simulink model "all_in_one"  (R2022b)
settings: Solver=VariableStepAuto  StartTime=0.0  StopTime=10.0  RelTol=1e-3
settings Model: Creator=GROUP LAPTOPS  LastModifiedBy=GROUP LAPTOPS
settings OptimizationCC: DefaultParameterBehavior=Inlined  EnhancedBackFolding=on  PassReuseOutputArgsThreshold=0  OptimizeBlockOrder=speed  DifferentSizesBufferReuse=on  OptimizationCustomize=off
settings DebuggingCC: ParameterTunabilityLossMsg=error
settings HardwareCC: TargetBitPerPointer=64  TargetBitPerSizeT=64  TargetBitPerPtrDiffT=64  TargetLongLongMode=on  TargetIntDivRoundTo=Zero  TargetEndianess=LittleEndian  TargetWordSize=64  TargetHWDeviceType=MATLAB Host  ProdEqTarget=off
settings SFSimCC: MATLABDynamicMemAlloc=off
settings RTWCC: Description=Rapid Simulation Target  SystemTargetFile=rsim.tlc  TemplateMakefile=rsim_default_tmf  GenerateReport=on
settings CodeAppCC: ForceParamTrailComments=on  OperatorAnnotations=on
settings RSimTargetCC: TargetLangStandard=C99 (ISO)  OptimizeReductions=off

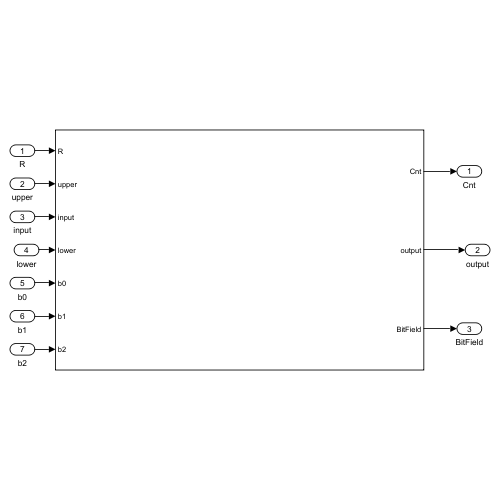
[thumbnail: Simulink's stored preview of the top-level diagram]
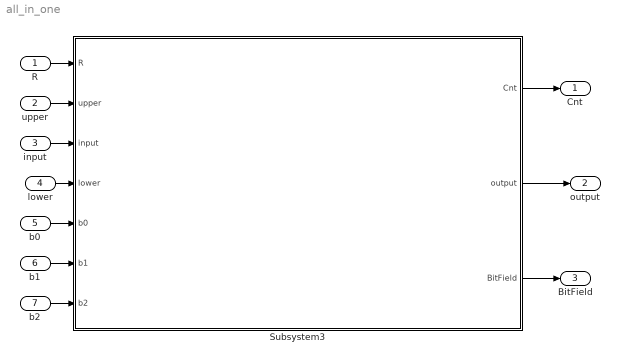
== system all_in_one ==
  R : Inport
  upper : Inport  Port=2
  input : Inport  Port=3
  lower : Inport  Port=4
  b0 : Inport  Port=5
  b1 : Inport  Port=6
  b2 : Inport  Port=7
  Subsystem3 : Subsystem
  Cnt : Outport
  output : Outport  Port=2
  BitField : Outport  Port=3
  wires:
  R/1 -> Subsystem3/1(R)
  upper/1 -> Subsystem3/2(upper)
  input/1 -> Subsystem3/3(input)
  lower/1 -> Subsystem3/4(lower)
  b2/1 -> Subsystem3/7(b2)
  b1/1 -> Subsystem3/6(b1)
  b0/1 -> Subsystem3/5(b0)
  Subsystem3/1(Cnt) -> Cnt/1
  Subsystem3/3(BitField) -> BitField/1
  Subsystem3/2(output) -> output/1

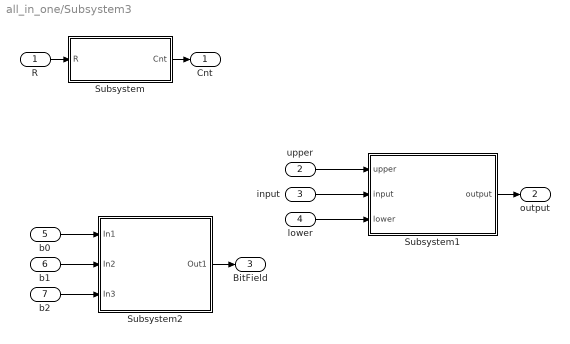
== system all_in_one/Subsystem3 ==
  R : Inport
  upper : Inport  Port=2
  input : Inport  Port=3
  lower : Inport  Port=4
  b0 : Inport  Port=5
  b1 : Inport  Port=6
  b2 : Inport  Port=7
  Subsystem : Subsystem
  Subsystem1 : Subsystem
  Subsystem2 : Subsystem
  Cnt : Outport
  output : Outport  Port=2
  BitField : Outport  Port=3
  wires:
  b0/1 -> Subsystem2/1(In1)
  Subsystem2/1(Out1) -> BitField/1
  upper/1 -> Subsystem1/1(upper)
  Subsystem1/1(output) -> output/1
  R/1 -> Subsystem/1(R)
  input/1 -> Subsystem1/2(input)
  Subsystem/1(Cnt) -> Cnt/1
  b1/1 -> Subsystem2/2(In2)
  b2/1 -> Subsystem2/3(In3)
  lower/1 -> Subsystem1/3(lower)

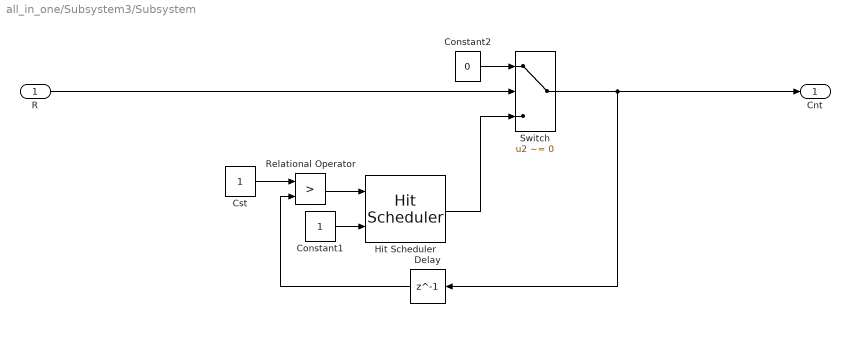
== system all_in_one/Subsystem3/Subsystem ==
  R : Inport
  Constant1 : Constant
  Constant2 : Constant  Value=0
  Cst : Constant
  Delay : Delay  DelayLength=1  InitialCondition=0
  Hit Scheduler : HitScheduler
  Relational Operator : RelationalOperator  Operator=>  OutDataTypeStr=boolean  RndMeth=Simplest  InputSameDT=off
  Switch : Switch  Criteria=u2 ~= 0  SaturateOnIntegerOverflow=off  InputSameDT=off
  Cnt : Outport
  wires:
  Relational Operator/1 -> Hit Scheduler/1
  Constant1/1 -> Hit Scheduler/2
  Switch/1 -> Cnt/1, Delay/1
  Delay/1 -> Relational Operator/2
  Cst/1 -> Relational Operator/1
  Constant2/1 -> Switch/1
  Hit Scheduler/1 -> Switch/3
  R/1 -> Switch/2

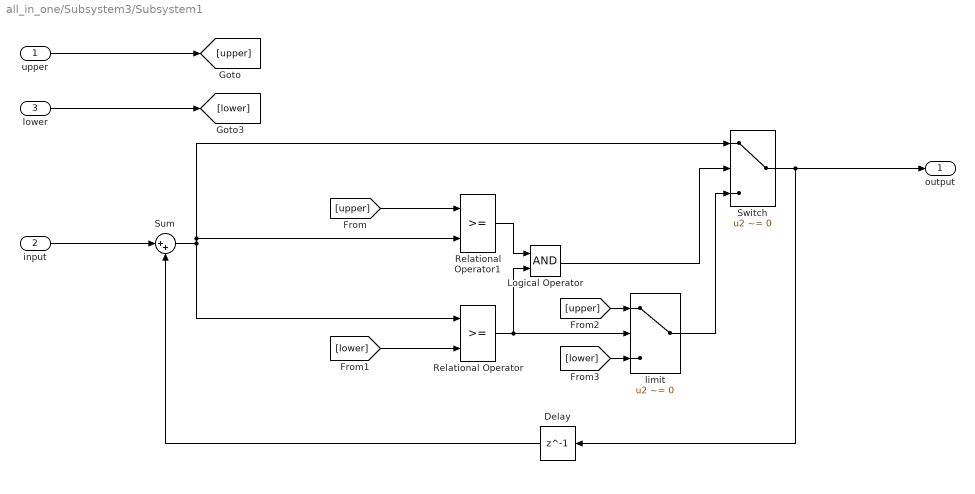
== system all_in_one/Subsystem3/Subsystem1 ==
  upper : Inport
  input : Inport  Port=2
  lower : Inport  Port=3
  Delay : Delay  DelayLength=1  InitialCondition=0
  Logical Operator : Logic  AllPortsSameDT=off  OutDataTypeStr=boolean
  Relational Operator : RelationalOperator  OutDataTypeStr=boolean  RndMeth=Simplest  InputSameDT=off
  Relational Operator1 : RelationalOperator  OutDataTypeStr=boolean  RndMeth=Simplest  InputSameDT=off
  Sum : Sum  Inputs=|++
  Switch : Switch  Criteria=u2 ~= 0  ZeroCross=off  SaturateOnIntegerOverflow=off  InputSameDT=off
  limit : Switch  Criteria=u2 ~= 0  ZeroCross=off  SaturateOnIntegerOverflow=off  InputSameDT=off
  output : Outport
  wires:
  [lower] -> Relational Operator/2
  lower/1 -> [lower]
  [lower] -> limit/3
  Logical Operator/1 -> Switch/2
  [upper] -> Relational Operator1/1
  Relational Operator/1 -> Logical Operator/2, limit/2
  [upper] -> limit/1
  input/1 -> Sum/1
  Switch/1 -> Delay/1, output/1
  Delay/1 -> Sum/2
  Relational Operator1/1 -> Logical Operator/1
  upper/1 -> [upper]
  Sum/1 -> Relational Operator1/2, Switch/1, Relational Operator/1
  limit/1 -> Switch/3

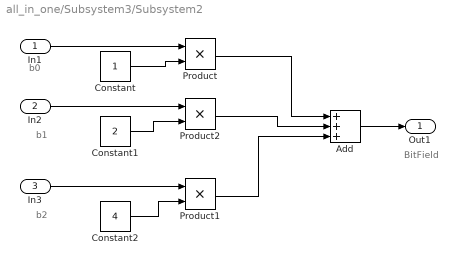
== system all_in_one/Subsystem3/Subsystem2 ==
  note: BitField
  note: b2
  note: b0
  note: b1
  In1 : Inport
  In2 : Inport  Port=2
  In3 : Inport  Port=3
  Add : Sum  Inputs=+++
  Constant : Constant
  Constant1 : Constant  Value=2
  Constant2 : Constant  Value=4
  Product : Product
  Product1 : Product
  Product2 : Product
  Out1 : Outport
  wires:
  Product/1 -> Add/1
  In1/1 -> Product/1
  Constant1/1 -> Product2/2
  Constant2/1 -> Product1/2
  Product2/1 -> Add/2
  Product1/1 -> Add/3
  In2/1 -> Product2/1
  Add/1 -> Out1/1
  In3/1 -> Product1/1
  Constant/1 -> Product/2
